simulink model "autocontroller_origin"  (R2024b)
settings: Solver=VariableStepAuto  StartTime=0.0  StopTime=10.0  RelTol=1e-3
undefined symbols (not defined in the file): control, controlParams, ControlSampleTime, Cruise_a, flightState, FWControlParams, FWTrimSpeed, uavParam, w_trim
libraries: slpidlib x21, simulink x8
(part 1 of 3)
settings Model: Creator=USER  LastModifiedBy=USER

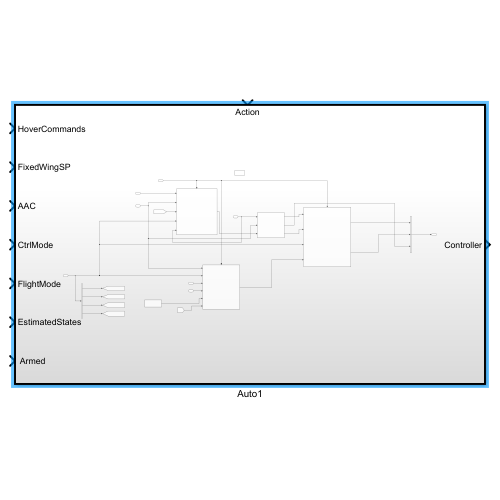
[thumbnail: Simulink's stored preview of the top-level diagram]
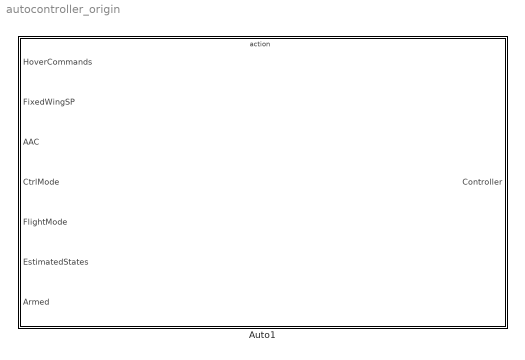
== system autocontroller_origin ==
  Auto1 : Subsystem  TreatAsAtomicUnit=on

== system autocontroller_origin/Auto1 ==
  HoverCommands : Inport  OutDataTypeStr=Bus: HoverSPBus
  FixedWingSP : Inport  Port=2
  AAC : Inport  Port=3
  CtrlMode : Inport  Port=4
  FlightMode : Inport  Port=5
  EstimatedStates : Inport  Port=6
  " Armed" : Inport  Port=7
  Action Port : ActionPort
  Blend Scheduler : Subsystem
  Bus Creator : BusCreator  Inputs=3  OutDataTypeStr=Bus: controller
  Bus Selector2 : BusSelector  OutputSignals=inTransition,TransitionCondition,BackTransitionCondition,TransitionStep
  Fixed Wing Controller : Subsystem  TreatAsAtomicUnit=on  VariantControl=Fixed Wing Controller
  Manual Control : Subsystem
  Multicopter Controller : Subsystem  TreatAsAtomicUnit=on
  Scheduler : Subsystem  SystemSampleTime=0.005
  Controller : Outport
  wires:
  Scheduler/1(MotorActuatorCommands) -> Bus Creator/1  "MotorActuatorCommands"
  Manual Control/1(AERT) -> Fixed Wing Controller/5(AERT)
  Scheduler/2(CtrlSurfaceCommands) -> Bus Creator/2  "CtrlSurfaceCommands"
  Fixed Wing Controller/1(Actuator) -> Scheduler/4(FixedWingActuators)
  Blend Scheduler/2(alpha) -> Bus Creator/3  "a"
  Multicopter Controller/1(MixerCommands) -> Blend Scheduler/3(MixerCommands)
  AAC/1 -> Fixed Wing Controller/3(AAC SP)
  FixedWingSP/1 -> Fixed Wing Controller/4(FixedWingSP)
  [InTransition] -> Multicopter Controller/3(InTransition)
  " Armed"/1 -> Fixed Wing Controller/Enable, Scheduler/Enable, Multicopter Controller/Enable
  HoverCommands/1 -> Multicopter Controller/1(Hover Commands)
  EstimatedStates/1 -> Fixed Wing Controller/1(States), Blend Scheduler/2(States), Multicopter Controller/2(States)
  FlightMode/1 -> Multicopter Controller/5(FlightMode), Blend Scheduler/1(FlightMode)
  Bus Selector2/2 -> [TransitionDone]  "<TransitionCondition>"
  CtrlMode/1 -> Bus Selector2/1, Scheduler/3(CtrlMode), Multicopter Controller/4(CtrlMode), Fixed Wing Controller/2(Control Mode)
  Bus Selector2/1 -> [InTransition]  "<inTransition>"
  Bus Selector2/3 -> [BackTransitionDone]  "<BackTransitionCondition>"
  Bus Creator/1 -> Controller/1
  Blend Scheduler/3(FlightState) -> Scheduler/2(FlightState)
  [InTransition] -> Fixed Wing Controller/6(In1)
  Bus Selector2/4 -> [TransitionStep]  "<TransitionStep>"
  Blend Scheduler/1(MotorCommands) -> Scheduler/1(MotorCommands)

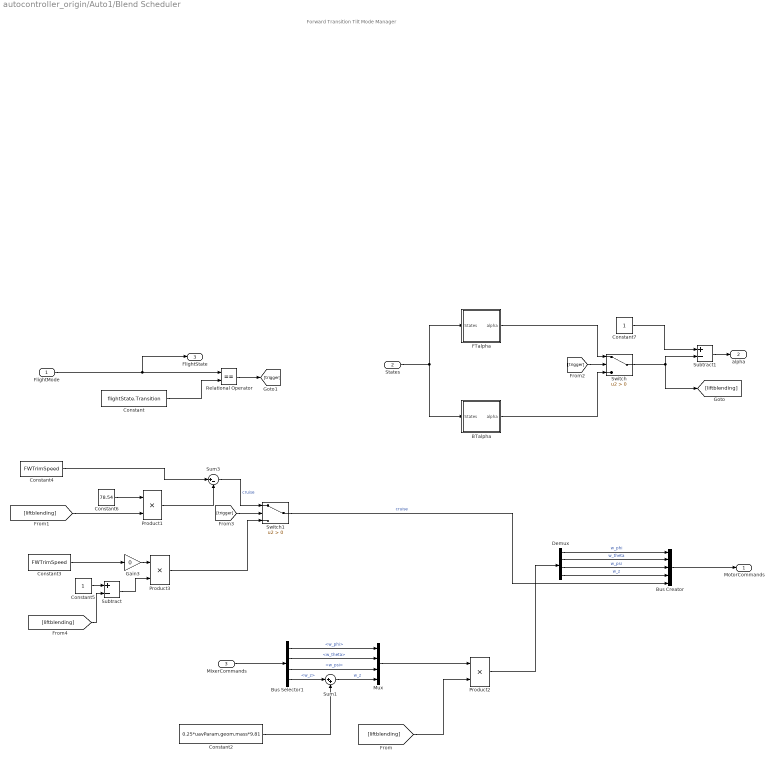
== system autocontroller_origin/Auto1/Blend Scheduler ==
  note: Forward Transition Tilt Mode Manager
  FlightMode : Inport
  States : Inport  Port=2
  MixerCommands : Inport  Port=3
  BTalpha : Subsystem  TreatAsAtomicUnit=on
  Bus Creator : BusCreator  Inputs=5
  Bus Selector1 : BusSelector  OutputSignals=w_phi,w_theta,w_psi,w_z
  Constant : Constant  Value=flightState.Transition
  Constant2 : Constant  Value=0.25*uavParam.geom.mass*9.81
  Constant3 : Constant  Value=FWTrimSpeed
  Constant4 : Constant  Value=FWTrimSpeed
  Constant5 : Constant
  Constant6 : Constant  Value=78.54
  Constant7 : Constant
  Demux : Demux
  FTalpha : Subsystem
  Gain3 : Gain  Gain=0
  Mux : Mux
  Product1 : Product
  Product2 : Product
  Product3 : Product
  Relational Operator : RelationalOperator  Operator===  OutDataTypeStr=boolean  RndMeth=Simplest  InputSameDT=off
  Subtract : Sum  Inputs=+-
  Subtract1 : Sum  Inputs=+-
  Sum1 : Sum  Inputs=|++
  Sum3 : Sum  Inputs=|+-
  Switch : Switch  Criteria=u2 > Threshold  SaturateOnIntegerOverflow=off  InputSameDT=off
  Switch1 : Switch  Criteria=u2 > Threshold  SaturateOnIntegerOverflow=off  InputSameDT=off
  MotorCommands : Outport
  alpha : Outport  Port=2
  FlightState : Outport  Port=3
  wires:
  FlightMode/1 -> Relational Operator/1, FlightState/1
  Relational Operator/1 -> [trigger]
  Bus Selector1/4 -> Sum1/1  "<w_z>"
  Constant2/1 -> Sum1/2
  [liftblending] -> Product2/2
  Mux/1 -> Product2/1
  MixerCommands/1 -> Bus Selector1/1
  Bus Selector1/1 -> Mux/1  "<w_phi>"
  Bus Selector1/2 -> Mux/2  "<w_theta>"
  Bus Selector1/3 -> Mux/3  "<w_psi>"
  Sum1/1 -> Mux/4  "w_z"
  Product2/1 -> Demux/1
  Demux/1 -> Bus Creator/1  "w_phi"
  Demux/2 -> Bus Creator/2  "w_theta"
  Demux/3 -> Bus Creator/3  "w_psi"
  Demux/4 -> Bus Creator/4  "w_z"
  Bus Creator/1 -> MotorCommands/1
  Constant6/1 -> Product1/1
  States/1 -> FTalpha/1(States), BTalpha/1(States)
  Switch/1 -> [liftblending], Subtract1/2
  FTalpha/1(alpha) -> Switch/1
  BTalpha/1(alpha) -> Switch/3
  [trigger] -> Switch/2
  Product1/1 -> Sum3/2
  Sum3/1 -> Switch1/1  "cruise"
  [trigger] -> Switch1/2
  Switch1/1 -> Bus Creator/5  "cruise"
  Constant3/1 -> Gain3/1
  Gain3/1 -> Product3/1
  Constant5/1 -> Subtract/1
  [liftblending] -> Subtract/2
  Subtract/1 -> Product3/2
  Product3/1 -> Switch1/3
  Constant7/1 -> Subtract1/1
  Subtract1/1 -> alpha/1
  Constant/1 -> Relational Operator/2
  [liftblending] -> Product1/2
  Constant4/1 -> Sum3/1

== system autocontroller_origin/Auto1/Fixed Wing Controller ==
  States : Inport
  Control Mode : Inport  Port=2
  AAC SP : Inport  Port=3  OutDataTypeStr=Bus: AAC
  FixedWingSP : Inport  Port=4  OutDataTypeStr=Bus: FixedWingCommandBus
  AERT : Inport  Port=5
  In1 : Inport  Port=6
  Actuator Armed : EnablePort
  Subsystem : Subsystem
  Actuator : Outport
  wires:
  States/1 -> Subsystem/1(States)
  Control Mode/1 -> Subsystem/2(Control Mode)
  AAC SP/1 -> Subsystem/3(AAC SP)
  Subsystem/1(Actuator) -> Actuator/1
  AERT/1 -> Subsystem/5(AERT)
  FixedWingSP/1 -> Subsystem/4(FixedWingSP)
  In1/1 -> Subsystem/6(Intransition)

== system autocontroller_origin/Auto1/Manual Control ==
  Bus Creator : BusCreator  Inputs=4
  Constant{,1..3} (4 alike) : Constant  Value=0  SampleTime=-1
  AERT : Outport
  wires:
  Constant/1 -> Bus Creator/1  "aileron"
  Constant1/1 -> Bus Creator/2  "throttle"
  Constant2/1 -> Bus Creator/3  "elevator"
  Constant3/1 -> Bus Creator/4  "rudder"
  Bus Creator/1 -> AERT/1

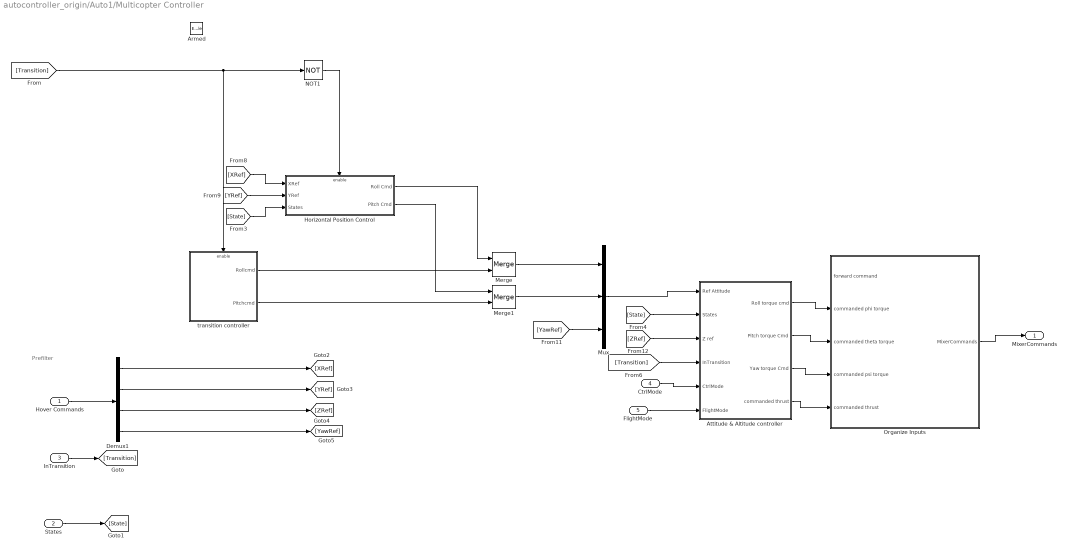
== system autocontroller_origin/Auto1/Multicopter Controller ==
  note: Prefilter
  Hover Commands : Inport  OutDataTypeStr=Bus: HoverSPBus
  States : Inport  Port=2
  InTransition : Inport  Port=3
  CtrlMode : Inport  Port=4
  FlightMode : Inport  Port=5
  " Armed" : EnablePort
  Attitude & Altitude controller : Subsystem
  Demux1 : Demux
  Horizontal Position Control : Subsystem  TreatAsAtomicUnit=on
  Merge : Merge
  Merge1 : Merge
  Mux : Mux  Inputs=3
  NOT1 : Logic  Operator=NOT  IconShape=distinctive  AllPortsSameDT=off  OutDataTypeStr=boolean
  Organize Inputs : Subsystem
  transition controller : Subsystem
  MixerCommands : Outport
  wires:
  Organize Inputs/1(MixerCommands) -> MixerCommands/1
  Demux1/1 -> [XRef]
  [State] -> Horizontal Position Control/3(States)
  Demux1/3 -> [ZRef]
  NOT1/1 -> Horizontal Position Control/Enable
  [XRef] -> Horizontal Position Control/1(XRef)
  [YRef] -> Horizontal Position Control/2(YRef)
  InTransition/1 -> [Transition]
  States/1 -> [State]
  Hover Commands/1 -> Demux1/1
  Demux1/4 -> [YawRef]
  Mux/1 -> Attitude & Altitude controller/1(Ref Attitude)
  [State] -> Attitude & Altitude controller/2(States)
  [ZRef] -> Attitude & Altitude controller/3(Z ref)
  [Transition] -> Attitude & Altitude controller/4(InTransition)
  Attitude & Altitude controller/1(Roll torque cmd) -> Organize Inputs/2(commanded phi torque)
  Attitude & Altitude controller/2(Pitch torque Cmd) -> Organize Inputs/3(commanded theta torque)
  Attitude & Altitude controller/4(commanded thrust) -> Organize Inputs/5(commanded thrust)
  FlightMode/1 -> Attitude & Altitude controller/6(FlightMode)
  Attitude & Altitude controller/3(Yaw torque Cmd) -> Organize Inputs/4(commanded psi torque)
  [Transition] -> NOT1/1, transition controller/Enable
  [YawRef] -> Mux/3
  Demux1/2 -> [YRef]
  Merge/1 -> Mux/1
  Merge1/1 -> Mux/2
  transition controller/1(Rollcmd) -> Merge/2
  transition controller/2(Pitchcmd) -> Merge1/2
  Horizontal Position Control/1(Roll Cmd) -> Merge/1
  Horizontal Position Control/2(Pitch Cmd) -> Merge1/1
  CtrlMode/1 -> Attitude & Altitude controller/5(CtrlMode)

== system autocontroller_origin/Auto1/Scheduler ==
  MotorCommands : Inport
  FlightState : Inport  Port=2  OutDataTypeStr=Enum: flightState
  CtrlMode : Inport  Port=3
  FixedWingActuators : Inport  Port=4
  " Armed" : EnablePort
  FixedWingScheduler : Subsystem
  Subsystem : Subsystem
  MotorActuatorCommands : Outport  OutputWhenDisabled=reset  InitialOutput=0
  CtrlSurfaceCommands : Outport  Port=2  OutDataTypeStr=Bus: FixedWingCtrlBus  OutputWhenDisabled=reset  InitialOutput=0  VectorParamsAs1DForOutWhenUnconnected=off
  wires:
  FixedWingScheduler/1(ActuatorControls) -> CtrlSurfaceCommands/1, Subsystem/2(FixedWingActuators)
  FlightState/1 -> Subsystem/1(FlightState), FixedWingScheduler/1(FlightState)
  Subsystem/1(ActuatorControls) -> MotorActuatorCommands/1
  MotorCommands/1 -> Subsystem/4(MotorCommands)
  FixedWingActuators/1 -> FixedWingScheduler/2(FixedWingActuators)
  CtrlMode/1 -> Subsystem/3(CtrlMode)

== system autocontroller_origin/Auto1/Blend Scheduler/BTalpha ==
  States : Inport
  Bus Selector : BusSelector  OutputSignals=airspeed
  Constant : Constant  Value=65
  Gain : Gain  Gain=1/20
  Saturation : Saturate  UpperLimit=1  LowerLimit=0
  Subtract : Sum  Inputs=+-
  alpha : Outport
  wires:
  Constant/1 -> Subtract/1
  Subtract/1 -> Gain/1
  Gain/1 -> Saturation/1
  Saturation/1 -> alpha/1
  States/1 -> Bus Selector/1
  Bus Selector/1 -> Subtract/2  "<airspeed>"

== system autocontroller_origin/Auto1/Blend Scheduler/FTalpha ==
  States : Inport
  1-a : Sum  Inputs=+-
  Bus Selector : BusSelector  OutputSignals=airspeed
  Constant3 : Constant  Value=35
  Constant5 : Constant  Value=Cruise_a
  Gain3 : Gain  Gain=1/10
  Saturation1 : Saturate  UpperLimit=10  LowerLimit=0
  Sum2 : Sum  Inputs=|+-
  alpha : Outport
  wires:
  1-a/1 -> alpha/1
  Bus Selector/1 -> Sum2/1  "<airspeed>"
  Gain3/1 -> 1-a/2
  Sum2/1 -> Saturation1/1
  Saturation1/1 -> Gain3/1
  Constant3/1 -> Sum2/2
  States/1 -> Bus Selector/1
  Constant5/1 -> 1-a/1

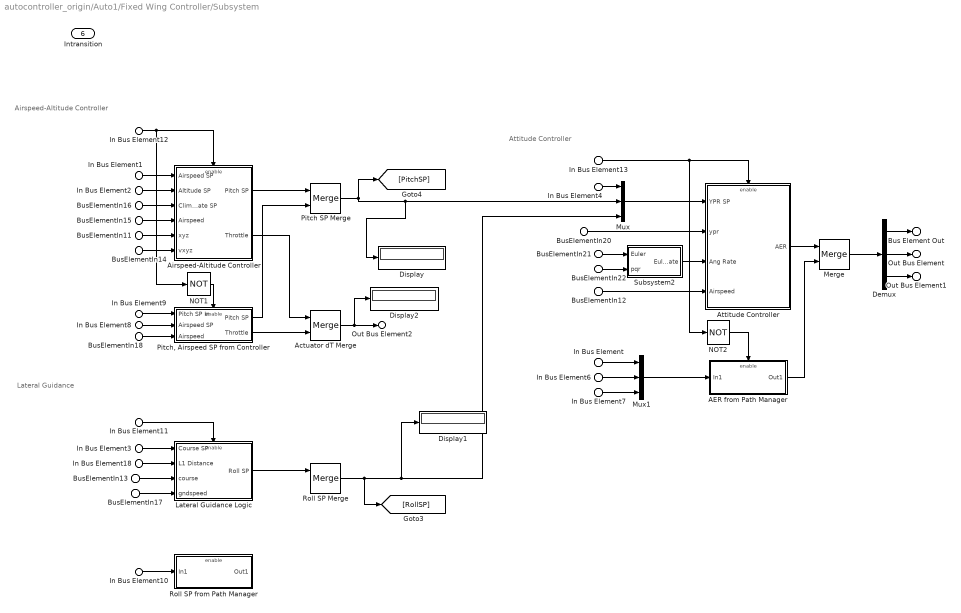
== system autocontroller_origin/Auto1/Fixed Wing Controller/Subsystem ==
  note: Airspeed-Altitude Controller
  note: Lateral Guidance
  note: Attitude Controller
  BusElementIn11 : Inport  PortName=States  Element=Xe
  BusElementIn12 : Inport  PortName=States  Element=airspeed
  BusElementIn15 : Inport  PortName=States  Element=airspeed
  BusElementIn18 : Inport  PortName=States  Element=airspeed
  BusElementIn13 : Inport  PortName=States  Element=course
  BusElementIn16 : Inport  PortName=States  Element=course
  BusElementIn14 : Inport  PortName=States  Element=Ve_ground
  BusElementIn17 : Inport  PortName=States  Element=gndspeed
  BusElementIn20 : Inport  PortName=States  Element=YPR
  BusElementIn21 : Inport  PortName=States  Element=Euler
  BusElementIn22 : Inport  PortName=States  Element=pqr
  In Bus Element11 : Inport  Port=2  PortName=Control Mode  Element=lateralGuidance
  In Bus Element12 : Inport  Port=2  PortName=Control Mode  Element=airspeedAltitude
  In Bus Element13 : Inport  Port=2  PortName=Control Mode  Element=attitude
  In Bus Element1 : Inport  Port=3  PortName=AAC SP  Element=airspeed
  In Bus Element2 : Inport  Port=3  PortName=AAC SP  Element=altitude
  In Bus Element18 : Inport  Port=3  PortName=AAC SP  Element=L1
  In Bus Element3 : Inport  Port=3  PortName=AAC SP  Element=course
  In Bus Element4 : Inport  Port=4  PortName=FixedWingSP  Element=yaw
  In Bus Element9 : Inport  Port=4  PortName=FixedWingSP  Element=pitch
  In Bus Element10 : Inport  Port=4  PortName=FixedWingSP  Element=roll
  In Bus Element8 : Inport  Port=4  PortName=FixedWingSP  Element=airspeed
  In Bus Element : Inport  Port=5  PortName=AERT  Element=aileron
  In Bus Element6 : Inport  Port=5  PortName=AERT  Element=elevator
  In Bus Element7 : Inport  Port=5  PortName=AERT  Element=rudder
  Intransition : Inport  Port=6
  AER from Path Manager : Subsystem  TreatAsAtomicUnit=on
  Actuator dT Merge : Merge
  Airspeed-Altitude Controller : Subsystem
  Attitude Controller : Subsystem
  Demux : Demux  Outputs=3
  Display : Display
  Display1 : Display
  Display2 : Display
  Lateral Guidance Logic : Subsystem
  Merge : Merge
  Mux : Mux  Inputs=3
  Mux1 : Mux  Inputs=3
  NOT1 : Logic  Operator=NOT  IconShape=distinctive  AllPortsSameDT=off  OutDataTypeStr=boolean
  NOT2 : Logic  Operator=NOT  IconShape=distinctive  AllPortsSameDT=off  OutDataTypeStr=boolean
  Pitch SP Merge : Merge
  "Pitch, Airspeed SP from Controller" : Subsystem  TreatAsAtomicUnit=on
  Roll SP Merge : Merge
  Roll SP from Path Manager : Subsystem  TreatAsAtomicUnit=on
  Subsystem2 : Subsystem
  Bus Element Out : Outport  PortName=Actuator  Element=dA
  Out Bus Element : Outport  PortName=Actuator  Element=dE
  Out Bus Element1 : Outport  PortName=Actuator  Element=dR
  Out Bus Element2 : Outport  PortName=Actuator  Element=dT
  wires:
  In Bus Element4/1 -> Mux/1
  Roll SP Merge/1 -> [RollSP], Display1/1, Mux/3
  BusElementIn18/1 -> "Pitch, Airspeed SP from Controller"/3(Airspeed)
  In Bus Element12/1 -> Airspeed-Altitude Controller/Enable, NOT1/1
  In Bus Element3/1 -> Lateral Guidance Logic/1(Course SP)
  Mux1/1 -> AER from Path Manager/1(In1)
  In Bus Element11/1 -> Lateral Guidance Logic/Enable
  Lateral Guidance Logic/1(Roll SP) -> Roll SP Merge/1
  In Bus Element7/1 -> Mux1/3
  Demux/2 -> Out Bus Element/1
  Demux/1 -> Bus Element Out/1
  In Bus Element9/1 -> "Pitch, Airspeed SP from Controller"/1(Pitch SP In)
  Merge/1 -> Demux/1
  In Bus Element18/1 -> Lateral Guidance Logic/2(L1 Distance)
  In Bus Element13/1 -> NOT2/1, Attitude Controller/Enable
  "Pitch, Airspeed SP from Controller"/1(Pitch SP) -> Pitch SP Merge/2
  BusElementIn14/1 -> Airspeed-Altitude Controller/6(vxyz)
  Pitch SP Merge/1 -> Display/1, Mux/2, [PitchSP]
  BusElementIn15/1 -> Airspeed-Altitude Controller/4(Airspeed)
  In Bus Element8/1 -> "Pitch, Airspeed SP from Controller"/2(Airspeed SP)
  BusElementIn13/1 -> Lateral Guidance Logic/3(course)
  Airspeed-Altitude Controller/2(Throttle) -> Actuator dT Merge/1
  BusElementIn16/1 -> Airspeed-Altitude Controller/3(Climb Rate SP)
  In Bus Element1/1 -> Airspeed-Altitude Controller/1(Airspeed SP)
  BusElementIn11/1 -> Airspeed-Altitude Controller/5(xyz)
  BusElementIn12/1 -> Attitude Controller/4(Airspeed)
  In Bus Element2/1 -> Airspeed-Altitude Controller/2(Altitude SP)
  BusElementIn20/1 -> Attitude Controller/2(ypr)
  Mux/1 -> Attitude Controller/1(YPR SP)
  Demux/3 -> Out Bus Element1/1
  BusElementIn21/1 -> Subsystem2/1(Euler)
  Subsystem2/1(Euler Rate) -> Attitude Controller/3(Ang Rate)
  "Pitch, Airspeed SP from Controller"/2(Throttle) -> Actuator dT Merge/2
  Airspeed-Altitude Controller/1(Pitch SP) -> Pitch SP Merge/1
  Attitude Controller/1(AER) -> Merge/1
  AER from Path Manager/1(Out1) -> Merge/2
  In Bus Element/1 -> Mux1/1
  In Bus Element10/1 -> Roll SP from Path Manager/1(In1)
  In Bus Element6/1 -> Mux1/2
  NOT2/1 -> AER from Path Manager/Enable
  BusElementIn22/1 -> Subsystem2/2(pqr)
  Actuator dT Merge/1 -> Display2/1, Out Bus Element2/1
  BusElementIn17/1 -> Lateral Guidance Logic/4(gndspeed)
  NOT1/1 -> "Pitch, Airspeed SP from Controller"/Enable

== system autocontroller_origin/Auto1/Multicopter Controller/Attitude & Altitude controller ==
  Ref Attitude : Inport
  States : Inport  Port=2
  Z ref : Inport  Port=3
  InTransition : Inport  Port=4
  CtrlMode : Inport  Port=5
  FlightMode : Inport  Port=6
  Altitude Control : Subsystem
  Bus Selector : BusSelector  OutputSignals=RC
  Compare To Constant : simulink/Logic and Bit Operations/Compare To Constant  relop=>  const=1700  OutDataTypeStr=boolean
  Derivative Gain : Subsystem  VariantControl=AttitudeControl==1
  Selector : Selector  InputPortWidth=10  IndexOptions=Index vector (dialog)  Indices=7  OutputSizes=1
  Roll torque cmd : Outport
  Pitch torque Cmd : Outport  Port=2
  Yaw torque Cmd : Outport  Port=3
  commanded thrust : Outport  Port=4
  wires:
  Altitude Control/1(commanded thrust) -> commanded thrust/1
  Derivative Gain/1(Roll torque cmd) -> Roll torque cmd/1
  InTransition/1 -> Altitude Control/3(InTransition)
  Derivative Gain/2(Pitch torque Cmd) -> Pitch torque Cmd/1
  States/1 -> Derivative Gain/2(States), Bus Selector/1, Altitude Control/1(States)
  Derivative Gain/3(Yaw torque Cmd) -> Yaw torque Cmd/1
  Z ref/1 -> Altitude Control/2(Z ref)
  FlightMode/1 -> Altitude Control/4(FlightMode)
  Ref Attitude/1 -> Derivative Gain/1(Ref Attitude)
  Selector/1 -> Compare To Constant/1
  Bus Selector/1 -> Selector/1  "<RC>"
  Compare To Constant/1 -> Altitude Control/Enable
  CtrlMode/1 -> Derivative Gain/3(CtrlMode), Altitude Control/5(CtrlMode)

== system autocontroller_origin/Auto1/Multicopter Controller/Horizontal Position Control ==
  note: Forward Motion is controlled using Tilt.
      | Lateral Motion occurs using roll.
  XRef : Inport
  YRef : Inport  Port=2
  States : Inport  Port=3
  Enable : EnablePort  ShowOutputPort=on
  Saturation : Saturate  UpperLimit=0.75  LowerLimit=-0.75
  Saturation1 : Saturate  UpperLimit=1  LowerLimit=-0.75
  Signal Conversion : SignalConversion  OverrideOpt=off
  Signal Conversion1 : SignalConversion  OverrideOpt=off
  XY Controller : Subsystem
  Roll Cmd : Outport
  Pitch Cmd : Outport  Port=2
  wires:
  XRef/1 -> XY Controller/1(X_ref)
  YRef/1 -> XY Controller/2(Y_ref)
  States/1 -> XY Controller/3(States)
  XY Controller/1(Forward cmd) -> Saturation1/1
  XY Controller/2(Sideward Cmd) -> Saturation/1
  Saturation1/1 -> Signal Conversion/1
  Saturation/1 -> Signal Conversion1/1
  Signal Conversion/1 -> Pitch Cmd/1
  Signal Conversion1/1 -> Roll Cmd/1
  Enable/1 -> XY Controller/Enable

== system autocontroller_origin/Auto1/Multicopter Controller/Organize Inputs ==
  forward command : Inport
  commanded phi torque : Inport  Port=2
  commanded theta torque : Inport  Port=3
  commanded psi torque : Inport  Port=4
  commanded thrust : Inport  Port=5
  Out Bus Element : Outport  PortName=MixerCommands  Element=w_phi
  Out Bus Element1 : Outport  PortName=MixerCommands  Element=w_theta
  Out Bus Element2 : Outport  PortName=MixerCommands  Element=w_psi
  Out Bus Element3 : Outport  PortName=MixerCommands  Element=w_z
  Out Bus Element4 : Outport  PortName=MixerCommands  Element=l_x
  wires:
  forward command/1 -> Out Bus Element4/1
  commanded phi torque/1 -> Out Bus Element/1  "phi"
  commanded theta torque/1 -> Out Bus Element1/1
  commanded psi torque/1 -> Out Bus Element2/1
  commanded thrust/1 -> Out Bus Element3/1

== system autocontroller_origin/Auto1/Multicopter Controller/transition controller ==
  Enable : EnablePort
  Constant : Constant  Value=0
  Constant1 : Constant  Value=0
  Rollcmd : Outport
  Pitchcmd : Outport  Port=2
  wires:
  Constant/1 -> Rollcmd/1
  Constant1/1 -> Pitchcmd/1

== system autocontroller_origin/Auto1/Scheduler/FixedWingScheduler ==
  note: C opyright 2024 The MathWorks, Inc.
  note: Fixed Wing Control Mixer
  FlightState : Inport
  FixedWingActuators : Inport  Port=2  OutDataTypeStr=Bus: FixedWingCtrlBus
  Merge : Merge  Inputs=4
  Switch Case : SwitchCase  CaseConditions={flightState.Hover, flightState.Transition, flightState.FixedWing,flightState.BackTransition}  ShowDefaultCase=off
  Switch Case Action Subsystem : Subsystem  TreatAsAtomicUnit=on
  Switch Case Action Subsystem1 : Subsystem  TreatAsAtomicUnit=on
  Switch Case Action Subsystem2 : Subsystem  TreatAsAtomicUnit=on
  Switch Case Action Subsystem3 : Subsystem  TreatAsAtomicUnit=on
  ActuatorControls : Outport
  wires:
  FlightState/1 -> Switch Case/1
  FixedWingActuators/1 -> Switch Case Action Subsystem2/1(FixedWingActuators), Switch Case Action Subsystem1/1(FixedWingActuators)
  Switch Case/3 -> Switch Case Action Subsystem2/Action
  Switch Case/2 -> Switch Case Action Subsystem1/Action
  Switch Case Action Subsystem3/1(FixedWingControls) -> Merge/4
  Merge/1 -> ActuatorControls/1
  Switch Case Action Subsystem1/1(FixedWingControls) -> Merge/2
  Switch Case/4 -> Switch Case Action Subsystem3/Action
  Switch Case Action Subsystem/1(FixedWingControls) -> Merge/1
  Switch Case/1 -> Switch Case Action Subsystem/Action
  Switch Case Action Subsystem2/1(FixedWingControls) -> Merge/3

== system autocontroller_origin/Auto1/Scheduler/Subsystem ==
  note: C opyright 2024 The MathWorks, Inc.
  note: Multicopter Control Mixer
  FlightState : Inport
  FixedWingActuators : Inport  Port=2
  CtrlMode : Inport  Port=3
  MotorCommands : Inport  Port=4
  Actuator To Voltage : Subsystem
  Merge : Merge  Inputs=4
  Switch Case : SwitchCase  CaseConditions={flightState.Hover, flightState.Transition, flightState.FixedWing,flightState.BackTransition}  ShowDefaultCase=off
  Switch Case Action Subsystem : Subsystem  TreatAsAtomicUnit=on
  Switch Case Action Subsystem1 : Subsystem  TreatAsAtomicUnit=on
  Switch Case Action Subsystem2 : Subsystem  TreatAsAtomicUnit=on
  Switch Case Action Subsystem3 : Subsystem  TreatAsAtomicUnit=on
  ActuatorControls : Outport  OutDataTypeStr=Bus: FCCData
  wires:
  Switch Case/4 -> Switch Case Action Subsystem3/Action
  MotorCommands/1 -> Switch Case Action Subsystem3/1(MixerCommands), Switch Case Action Subsystem/1(MixerCommands), Switch Case Action Subsystem1/1(MixerCommands)
  FlightState/1 -> Switch Case/1
  Switch Case Action Subsystem3/1(Actuator) -> Merge/4
  FixedWingActuators/1 -> Switch Case Action Subsystem2/1(FixedWingCtrlBus)
  Switch Case/3 -> Switch Case Action Subsystem2/Action
  Switch Case/2 -> Switch Case Action Subsystem1/Action
  Switch Case Action Subsystem1/1(Actuator) -> Merge/2
  Switch Case/1 -> Switch Case Action Subsystem/Action
  Switch Case Action Subsystem2/1(Actuator) -> Merge/3
  Switch Case Action Subsystem/1(Actuator) -> Merge/1
  Merge/1 -> Actuator To Voltage/2(Motor Commands)
  Actuator To Voltage/1(Actuator) -> ActuatorControls/1
  CtrlMode/1 -> Actuator To Voltage/1(CtrlMode)

== system autocontroller_origin/Auto1/Fixed Wing Controller/Subsystem/AER from Path Manager ==
  In1 : Inport
  Enable : EnablePort
  Out1 : Outport
  wires:
  In1/1 -> Out1/1

== system autocontroller_origin/Auto1/Fixed Wing Controller/Subsystem/Airspeed-Altitude Controller ==
  note: Airspeed and altitude are controlled independently
      | by ignoring their coupled dynamics.
  Airspeed SP : Inport
  Altitude SP : Inport  Port=2
  Climb Rate SP : Inport  Port=3
  Airspeed : Inport  Port=4
  xyz : Inport  Port=5
  vxyz : Inport  Port=6
  Control Mode : EnablePort  ShowOutputPort=on
  Airspeed Controller : slpidlib/PID Controller  Controller=PID  Form=Parallel  TimeDomain=Discrete-time  UseExternalTs=off  SampleTime=ControlSampleTime  IntegratorMethod=Trapezoidal  FilterMethod=Forward Euler  ControllerParametersSource=internal  P=FWControlParams.P_AIRSPD  I=FWControlParams.I_AIRSPD  UseKiTs=off  D=FWControlParams.D_AIRSPD  UseExternalDerivativeSource=off  N=FWControlParams.N_AIRSPD  UseFilter=on  TunerSelectOption=Transfer Function Based (PID Tuner App)  InitialConditionSource=internal  InitialConditionForIntegrator=0  InitialConditionForFilter=0  DifferentiatorICPrevScaledInput=0  ExternalReset=none  TrackingMode=off  Kt=1  LimitOutput=off  SatLimitsSource=internal  UpperSaturationLimit=Inf  LowerSaturationLimit=0  LinearizeAsGain=on  AntiWindupMode=clamping  Kb=1  LimitIntegrator=off  UpperIntegratorSaturationLimit=inf  LowerIntegratorSaturationLimit=-inf  POutMin=[]  POutMax=[]  IOutMin=[]  IOutMax=[]  DOutMin=[]  DOutMax=[]  NOutMin=[]  NOutMax=[]  SumOutMin=[]  SumOutMax=[]  SaturationOutMin=[]  SaturationOutMax=[]  PParamMin=[]  PParamMax=[]  IParamMin=[]  IParamMax=[]  DParamMin=[]  DParamMax=[]  NParamMin=[]  NParamMax=[]  KbParamMin=[]  KbParamMax=[]  KtParamMin=[]  KtParamMax=[]  KbOutMin=[]  KbOutMax=[]  KtOutMin=[]  KtOutMax=[]  IntegratorOutMin=[]  IntegratorOutMax=[]  FilterOutMin=[]  FilterOutMax=[]  SumI1OutMin=[]  SumI1OutMax=[]  SumI2OutMin=[]  SumI2OutMax=[]  SumI3OutMin=[]  SumI3OutMax=[]  SumI4OutMin=[]  SumI4OutMax=[]  SumDOutMin=[]  SumDOutMax=[]  DifferentiatorOutMin=[]  DifferentiatorOutMax=[]  FilterDiffOutCoefMin=[]  FilterDiffOutCoefMax=[]  ReciprocalOutMin=[]  ReciprocalOutMax=[]  SumDenOutMin=[]  SumDenOutMax=[]  SumNumOutMin=[]  SumNumOutMax=[]  DivideOutMin=[]  DivideOutMax=[]  UdiffTsProdOutMin=[]  UdiffTsProdOutMax=[]  NTsProdOutMin=[]  NTsProdOutMax=[]  UintegralTsProdOutMin=[]  UintegralTsProdOutMax=[]  UngainTsProdOutMin=[]  UngainTsProdOutMax=[]  ClampingZeroOutDataTypeStr=Inherit: Inherit via back propagation  ClampingZeroOutMin=[]  ClampingZeroOutMax=[]  FilterDenConstantOutDataTypeStr=Inherit: Inherit via back propagation  FilterDenConstantOutMin=[]  FilterDenConstantOutMax=[]  PCopyOutDataTypeStr=Inherit: Inherit via back propagation  PCopyOutMin=[]  PCopyOutMax=[]  NCopyOutDataTypeStr=Inherit: Inherit via back propagation  NCopyOutMin=[]  NCopyOutMax=[]  IntegratorContinuousStateAttributes=''  IntegratorStateMustResolveToSignalObject=off  IntegratorRTWStateStorageClass=Auto  FilterContinuousStateAttributes=''  FilterStateMustResolveToSignalObject=off  FilterRTWStateStorageClass=Auto  ParallelPVariant=InternalParameters  IdealPVariant=Disabled  IVariant=InternalParameters  DVariant=InternalParameters  IntegratorVariant=Discrete  SatVariant=Disabled  AWVariant=Passthrough  PCopyVariant=Disabled  TRVariant=Disabled  FdbkBlocksVariant=Forward  IdealPFdbkVariant=Disabled  SatFdbkVariant=Disabled  DerivativeFilterVariant=ForwardEulerFilter  NVariant=InternalParameters  NCopyVariant=Disabled  FilterICVariant=InternalICsFilter  IntegratorICVariant=InternalICs  ExternalResetVariant=Disabled  TRSumVariant=Passthrough  SumFdbkVariant=Disabled  SumVariant=Sum_PID  TsampFilterVariant=InternalTs  TsampNgainVariant=Passthrough  TsampIntegralVariant=Disabled_SignalSpec  ExternalSaturationOutDataTypeStr=Inherit: Same as second input  DerivativeSourceVariant=ErrorSignal  PreIntVariant=InternalPreInt
  Altitude controller : Subsystem
  Climb Rate SP Merge : Merge
  Climb Rate SP from Guidance : Subsystem  TreatAsAtomicUnit=on
  Compare To Constant : simulink/Logic and Bit Operations/Compare To Constant  relop===  const=uint8(1)  OutDataTypeStr=boolean
  Compare To Constant1 : simulink/Logic and Bit Operations/Compare To Constant  relop===  const=uint8(2)  OutDataTypeStr=boolean
  Pitch SP Controller : Subsystem
  Sum1 : Sum  Inputs=|+-
  Pitch SP : Outport
  Throttle : Outport  Port=2
  wires:
  Airspeed SP/1 -> Sum1/1
  Sum1/1 -> Airspeed Controller/1
  Airspeed/1 -> Sum1/2
  Airspeed Controller/1 -> Throttle/1
  Altitude SP/1 -> Altitude controller/1(Alt SP)
  xyz/1 -> Altitude controller/2(xyz)
  vxyz/1 -> Pitch SP Controller/2(vxyz)
  Pitch SP Controller/1(Pitch SP) -> Pitch SP/1
  Control Mode/1 -> Compare To Constant1/1, Compare To Constant/1
  Compare To Constant/1 -> Altitude controller/Enable
  Compare To Constant1/1 -> Climb Rate SP from Guidance/Enable
  Altitude controller/1(Climb Rate SP) -> Climb Rate SP Merge/1
  Climb Rate SP from Guidance/1(Out1) -> Climb Rate SP Merge/2
  Climb Rate SP Merge/1 -> Pitch SP Controller/1(Climb Rate SP)
  Climb Rate SP/1 -> Climb Rate SP from Guidance/1(Climb Rate SP)

== system autocontroller_origin/Auto1/Fixed Wing Controller/Subsystem/Attitude Controller ==
  YPR SP : Inport
  ypr : Inport  Port=2
  Ang Rate : Inport  Port=3
  Airspeed : Inport  Port=4
  Enable : EnablePort  ShowOutputPort=on
  AER Merge : Merge
  Compare To Constant : simulink/Logic and Bit Operations/Compare To Constant  relop===  const=uint8(1)  OutDataTypeStr=boolean
  Compare To Constant1 : simulink/Logic and Bit Operations/Compare To Constant  relop===  const=uint8(2)  OutDataTypeStr=boolean
  Demux1 : Demux  Outputs=3
  Pitch Roll Controller : Subsystem
  Rudder Heading Controller : Subsystem
  AER : Outport
  wires:
  ypr/1 -> Rudder Heading Controller/2(YPR), Pitch Roll Controller/3(YPR)
  YPR SP/1 -> Demux1/1
  Enable/1 -> Compare To Constant1/1, Compare To Constant/1
  AER Merge/1 -> AER/1
  Compare To Constant/1 -> Pitch Roll Controller/Enable
  Pitch Roll Controller/1(AER) -> AER Merge/1
  Rudder Heading Controller/1(AER) -> AER Merge/2
  Demux1/1 -> Rudder Heading Controller/1(Yaw SP)
  Demux1/2 -> Pitch Roll Controller/1(Pitch SP)
  Demux1/3 -> Pitch Roll Controller/2(Roll SP)
  Ang Rate/1 -> Rudder Heading Controller/3(Ang Rate), Pitch Roll Controller/4(Ang Rate)
  Compare To Constant1/1 -> Rudder Heading Controller/Enable
  Airspeed/1 -> Pitch Roll Controller/5(Airspeed)

== system autocontroller_origin/Auto1/Fixed Wing Controller/Subsystem/Lateral Guidance Logic ==
  note: S. Park, J. Deyst, and J. P. How, "A New Nonlinear Guidance Logic for Trajectory Tracking," Proceedings of the AIAA Guidance, Navigation and Control Conference, Aug 2004. AIAA-2004-4900.
  Course SP : Inport
  L1 Distance : Inport  Port=2
  course : Inport  Port=3
  gndspeed : Inport  Port=4
  Enable : EnablePort
  Display{,1..3} (4 alike) : Display
  MATLAB Function : MATLAB Function  TreatAsAtomicUnit=on  SystemSampleTime=ControlSampleTime
  Terminator : Terminator
  Roll SP : Outport
  wires:
  course/1 -> Display1/1, MATLAB Function/2(course)
  MATLAB Function/2(rollSP) -> Roll SP/1
  MATLAB Function/1(lacc) -> Terminator/1
  gndspeed/1 -> Display2/1, MATLAB Function/3(groundSpeed)
  L1 Distance/1 -> Display3/1, MATLAB Function/4(L1)
  Course SP/1 -> Display/1, MATLAB Function/1(courseSP)

== system autocontroller_origin/Auto1/Fixed Wing Controller/Subsystem/Pitch, Airspeed SP from Controller ==
  Pitch SP In : Inport
  Airspeed SP : Inport  Port=2
  Airspeed : Inport  Port=3
  Enable : EnablePort
  Airspeed Controller : slpidlib/PID Controller  Controller=PID  Form=Parallel  TimeDomain=Discrete-time  UseExternalTs=off  SampleTime=ControlSampleTime  IntegratorMethod=Trapezoidal  FilterMethod=Forward Euler  ControllerParametersSource=internal  P=FWControlParams.P_AIRSPD  I=FWControlParams.I_AIRSPD*0  UseKiTs=off  D=FWControlParams.D_AIRSPD*0  UseExternalDerivativeSource=off  N=FWControlParams.N_AIRSPD  UseFilter=on  TunerSelectOption=Transfer Function Based (PID Tuner App)  InitialConditionSource=internal  InitialConditionForIntegrator=0  InitialConditionForFilter=0  DifferentiatorICPrevScaledInput=0  ExternalReset=none  TrackingMode=off  Kt=1  LimitOutput=off  SatLimitsSource=internal  UpperSaturationLimit=Inf  LowerSaturationLimit=0  LinearizeAsGain=on  AntiWindupMode=clamping  Kb=1  LimitIntegrator=off  UpperIntegratorSaturationLimit=inf  LowerIntegratorSaturationLimit=-inf  POutMin=[]  POutMax=[]  IOutMin=[]  IOutMax=[]  DOutMin=[]  DOutMax=[]  NOutMin=[]  NOutMax=[]  SumOutMin=[]  SumOutMax=[]  SaturationOutMin=[]  SaturationOutMax=[]  PParamMin=[]  PParamMax=[]  IParamMin=[]  IParamMax=[]  DParamMin=[]  DParamMax=[]  NParamMin=[]  NParamMax=[]  KbParamMin=[]  KbParamMax=[]  KtParamMin=[]  KtParamMax=[]  KbOutMin=[]  KbOutMax=[]  KtOutMin=[]  KtOutMax=[]  IntegratorOutMin=[]  IntegratorOutMax=[]  FilterOutMin=[]  FilterOutMax=[]  SumI1OutMin=[]  SumI1OutMax=[]  SumI2OutMin=[]  SumI2OutMax=[]  SumI3OutMin=[]  SumI3OutMax=[]  SumI4OutMin=[]  SumI4OutMax=[]  SumDOutMin=[]  SumDOutMax=[]  DifferentiatorOutMin=[]  DifferentiatorOutMax=[]  FilterDiffOutCoefMin=[]  FilterDiffOutCoefMax=[]  ReciprocalOutMin=[]  ReciprocalOutMax=[]  SumDenOutMin=[]  SumDenOutMax=[]  SumNumOutMin=[]  SumNumOutMax=[]  DivideOutMin=[]  DivideOutMax=[]  UdiffTsProdOutMin=[]  UdiffTsProdOutMax=[]  NTsProdOutMin=[]  NTsProdOutMax=[]  UintegralTsProdOutMin=[]  UintegralTsProdOutMax=[]  UngainTsProdOutMin=[]  UngainTsProdOutMax=[]  ClampingZeroOutDataTypeStr=Inherit: Inherit via back propagation  ClampingZeroOutMin=[]  ClampingZeroOutMax=[]  FilterDenConstantOutDataTypeStr=Inherit: Inherit via back propagation  FilterDenConstantOutMin=[]  FilterDenConstantOutMax=[]  PCopyOutDataTypeStr=Inherit: Inherit via back propagation  PCopyOutMin=[]  PCopyOutMax=[]  NCopyOutDataTypeStr=Inherit: Inherit via back propagation  NCopyOutMin=[]  NCopyOutMax=[]  IntegratorContinuousStateAttributes=''  IntegratorStateMustResolveToSignalObject=off  IntegratorRTWStateStorageClass=Auto  FilterContinuousStateAttributes=''  FilterStateMustResolveToSignalObject=off  FilterRTWStateStorageClass=Auto  ParallelPVariant=InternalParameters  IdealPVariant=Disabled  IVariant=InternalParameters  DVariant=InternalParameters  IntegratorVariant=Discrete  SatVariant=Disabled  AWVariant=Passthrough  PCopyVariant=Disabled  TRVariant=Disabled  FdbkBlocksVariant=Forward  IdealPFdbkVariant=Disabled  SatFdbkVariant=Disabled  DerivativeFilterVariant=ForwardEulerFilter  NVariant=InternalParameters  NCopyVariant=Disabled  FilterICVariant=InternalICsFilter  IntegratorICVariant=InternalICs  ExternalResetVariant=Disabled  TRSumVariant=Passthrough  SumFdbkVariant=Disabled  SumVariant=Sum_PID  TsampFilterVariant=InternalTs  TsampNgainVariant=Passthrough  TsampIntegralVariant=Disabled_SignalSpec  ExternalSaturationOutDataTypeStr=Inherit: Same as second input  DerivativeSourceVariant=ErrorSignal  PreIntVariant=InternalPreInt
  IC : InitialCondition  Value=0
  Sum1 : Sum  Inputs=|+-
  Pitch SP : Outport
  Throttle : Outport  Port=2
  wires:
  IC/1 -> Pitch SP/1
  Pitch SP In/1 -> IC/1
  Airspeed SP/1 -> Sum1/1
  Sum1/1 -> Airspeed Controller/1
  Airspeed/1 -> Sum1/2
  Airspeed Controller/1 -> Throttle/1

== system autocontroller_origin/Auto1/Fixed Wing Controller/Subsystem/Roll SP from Path Manager ==
  In1 : Inport
  Enable : EnablePort
  IC : InitialCondition  Value=0
  Out1 : Outport
  wires:
  In1/1 -> IC/1
  IC/1 -> Out1/1

== system autocontroller_origin/Auto1/Fixed Wing Controller/Subsystem/Subsystem2 ==
  Euler : Inport
  pqr : Inport  Port=2
  Demux : Demux  Outputs=3
  MATLAB Function : MATLAB Function  TreatAsAtomicUnit=on
  Terminator : Terminator
  Terminator1 : Terminator
  Euler Rate : Outport
  wires:
  Demux/1 -> MATLAB Function/1(phi)
  Demux/2 -> MATLAB Function/2(theta)
  MATLAB Function/1(y) -> Terminator1/1
  pqr/1 -> Euler Rate/1
  Euler/1 -> Demux/1
  Demux/3 -> Terminator/1

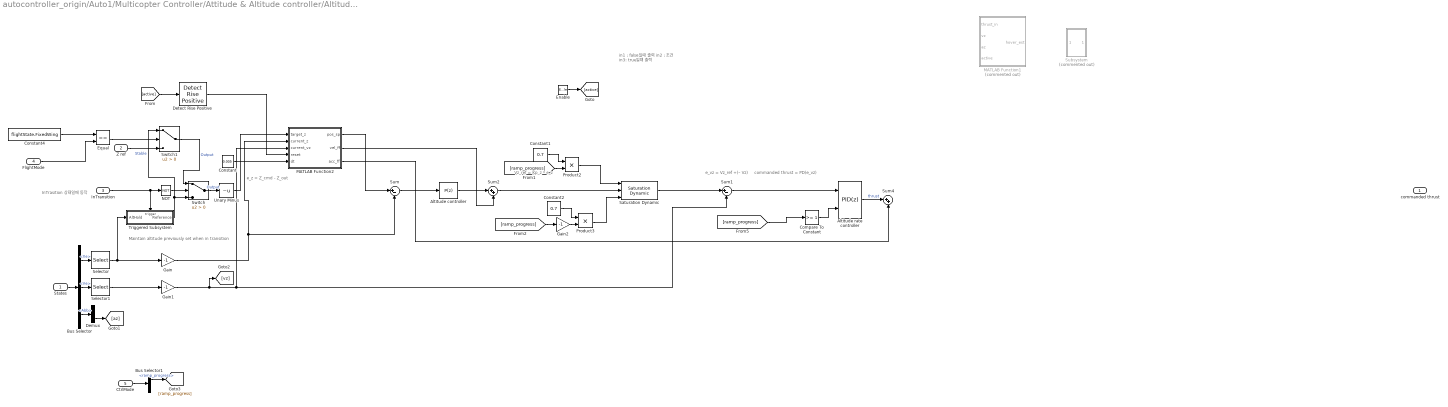
== system autocontroller_origin/Auto1/Multicopter Controller/Attitude & Altitude controller/Altitude Control ==
  note: commanded thrust = PD(e_vz)
  note: e_vz = Vz_ref +(– Vz)
  note: Vz_ref = Kp_z * e_z
  note: e_z = Z_cmd - Z_out
  note: in1 : false일때 출력
      | in2 : 조건
      | in3: true일떄 출력
  note: InTrasition 상태일때 동작
  note: Maintain altitude previously set when in transition
  States : Inport
  Z ref : Inport  Port=2
  InTransition : Inport  Port=3
  FlightMode : Inport  Port=4
  CtrlMode : Inport  Port=5
  Enable : EnablePort  StatesWhenEnabling=reset  ShowOutputPort=on
  Altitude controller : slpidlib/PID Controller  Controller=P  Form=Parallel  TimeDomain=Discrete-time  UseExternalTs=off  SampleTime=-1  IntegratorMethod=Forward Euler  FilterMethod=Forward Euler  ControllerParametersSource=internal  P=controlParams.P_Z  I=controlParams.I_Z  UseKiTs=off  D=controlParams.D_Z  UseExternalDerivativeSource=off  N=controlParams.N_Z  UseFilter=on  TunerSelectOption=Transfer Function Based (PID Tuner App)  InitialConditionSource=internal  InitialConditionForIntegrator=0  InitialConditionForFilter=0  DifferentiatorICPrevScaledInput=0  ExternalReset=none  TrackingMode=off  Kt=1  LimitOutput=on  SatLimitsSource=internal  UpperSaturationLimit=5  LowerSaturationLimit=-5  LinearizeAsGain=on  AntiWindupMode=none  Kb=1  LimitIntegrator=off  UpperIntegratorSaturationLimit=inf  LowerIntegratorSaturationLimit=-inf  POutMin=[]  POutMax=[]  IOutMin=[]  IOutMax=[]  DOutMin=[]  DOutMax=[]  NOutMin=[]  NOutMax=[]  SumOutMin=[]  SumOutMax=[]  SaturationOutMin=[]  SaturationOutMax=[]  PParamMin=[]  PParamMax=[]  IParamMin=[]  IParamMax=[]  DParamMin=[]  DParamMax=[]  NParamMin=[]  NParamMax=[]  KbParamMin=[]  KbParamMax=[]  KtParamMin=[]  KtParamMax=[]  KbOutMin=[]  KbOutMax=[]  KtOutMin=[]  KtOutMax=[]  IntegratorOutMin=[]  IntegratorOutMax=[]  FilterOutMin=[]  FilterOutMax=[]  SumI1OutMin=[]  SumI1OutMax=[]  SumI2OutMin=[]  SumI2OutMax=[]  SumI3OutMin=[]  SumI3OutMax=[]  SumI4OutMin=[]  SumI4OutMax=[]  SumDOutMin=[]  SumDOutMax=[]  DifferentiatorOutMin=[]  DifferentiatorOutMax=[]  FilterDiffOutCoefMin=[]  FilterDiffOutCoefMax=[]  ReciprocalOutMin=[]  ReciprocalOutMax=[]  SumDenOutMin=[]  SumDenOutMax=[]  SumNumOutMin=[]  SumNumOutMax=[]  DivideOutMin=[]  DivideOutMax=[]  UdiffTsProdOutMin=[]  UdiffTsProdOutMax=[]  NTsProdOutMin=[]  NTsProdOutMax=[]  UintegralTsProdOutMin=[]  UintegralTsProdOutMax=[]  UngainTsProdOutMin=[]  UngainTsProdOutMax=[]  ClampingZeroOutDataTypeStr=Inherit: Inherit via back propagation  ClampingZeroOutMin=[]  ClampingZeroOutMax=[]  FilterDenConstantOutDataTypeStr=Inherit: Inherit via back propagation  FilterDenConstantOutMin=[]  FilterDenConstantOutMax=[]  PCopyOutDataTypeStr=Inherit: Inherit via back propagation  PCopyOutMin=[]  PCopyOutMax=[]  NCopyOutDataTypeStr=Inherit: Inherit via back propagation  NCopyOutMin=[]  NCopyOutMax=[]  IntegratorContinuousStateAttributes=''  IntegratorStateMustResolveToSignalObject=off  IntegratorRTWStateStorageClass=Auto  FilterContinuousStateAttributes=''  FilterStateMustResolveToSignalObject=off  FilterRTWStateStorageClass=Auto  ParallelPVariant=InternalParameters  IdealPVariant=Disabled  IVariant=Disabled  DVariant=Disabled  IntegratorVariant=Disabled  SatVariant=Enabled  AWVariant=Disabled  PCopyVariant=Disabled  TRVariant=Disabled  FdbkBlocksVariant=Forward  IdealPFdbkVariant=Disabled  SatFdbkVariant=Disabled  DerivativeFilterVariant=Disabled  NVariant=Disabled  NCopyVariant=Disabled_SignalSpec  FilterICVariant=Disabled  IntegratorICVariant=Disabled  ExternalResetVariant=Disabled  TRSumVariant=Passthrough  SumFdbkVariant=Disabled  SumVariant=Passthrough_P  TsampFilterVariant=InternalTs  TsampNgainVariant=Passthrough  TsampIntegralVariant=Disabled_SignalSpec  ExternalSaturationOutDataTypeStr=Inherit: Same as second input  DerivativeSourceVariant=Disabled  PreIntVariant=InternalPreInt
  Altitude rate controller : slpidlib/PID Controller  Controller=PID  Form=Parallel  TimeDomain=Discrete-time  UseExternalTs=off  SampleTime=-1  IntegratorMethod=Forward Euler  FilterMethod=Forward Euler  ControllerParametersSource=internal  P=controlParams.P_VZ  I=controlParams.I_VZ  UseKiTs=off  D=controlParams.D_VZ  UseExternalDerivativeSource=off  N=controlParams.N_VZ  UseFilter=on  TunerSelectOption=Transfer Function Based (PID Tuner App)  InitialConditionSource=internal  InitialConditionForIntegrator=0  InitialConditionForFilter=0  DifferentiatorICPrevScaledInput=0  ExternalReset=rising  TrackingMode=off  Kt=1  LimitOutput=on  SatLimitsSource=internal  UpperSaturationLimit=2  LowerSaturationLimit=-2  LinearizeAsGain=on  AntiWindupMode=clamping  Kb=1  LimitIntegrator=on  UpperIntegratorSaturationLimit=2  LowerIntegratorSaturationLimit=-1.5  POutMin=[]  POutMax=[]  IOutMin=[]  IOutMax=[]  DOutMin=[]  DOutMax=[]  NOutMin=[]  NOutMax=[]  SumOutMin=[]  SumOutMax=[]  SaturationOutMin=[]  SaturationOutMax=[]  PParamMin=[]  PParamMax=[]  IParamMin=[]  IParamMax=[]  DParamMin=[]  DParamMax=[]  NParamMin=[]  NParamMax=[]  KbParamMin=[]  KbParamMax=[]  KtParamMin=[]  KtParamMax=[]  KbOutMin=[]  KbOutMax=[]  KtOutMin=[]  KtOutMax=[]  IntegratorOutMin=[]  IntegratorOutMax=[]  FilterOutMin=[]  FilterOutMax=[]  SumI1OutMin=[]  SumI1OutMax=[]  SumI2OutMin=[]  SumI2OutMax=[]  SumI3OutMin=[]  SumI3OutMax=[]  SumI4OutMin=[]  SumI4OutMax=[]  SumDOutMin=[]  SumDOutMax=[]  DifferentiatorOutMin=[]  DifferentiatorOutMax=[]  FilterDiffOutCoefMin=[]  FilterDiffOutCoefMax=[]  ReciprocalOutMin=[]  ReciprocalOutMax=[]  SumDenOutMin=[]  SumDenOutMax=[]  SumNumOutMin=[]  SumNumOutMax=[]  DivideOutMin=[]  DivideOutMax=[]  UdiffTsProdOutMin=[]  UdiffTsProdOutMax=[]  NTsProdOutMin=[]  NTsProdOutMax=[]  UintegralTsProdOutMin=[]  UintegralTsProdOutMax=[]  UngainTsProdOutMin=[]  UngainTsProdOutMax=[]  ClampingZeroOutDataTypeStr=Inherit: Inherit via back propagation  ClampingZeroOutMin=[]  ClampingZeroOutMax=[]  FilterDenConstantOutDataTypeStr=Inherit: Inherit via back propagation  FilterDenConstantOutMin=[]  FilterDenConstantOutMax=[]  PCopyOutDataTypeStr=Inherit: Inherit via back propagation  PCopyOutMin=[]  PCopyOutMax=[]  NCopyOutDataTypeStr=Inherit: Inherit via back propagation  NCopyOutMin=[]  NCopyOutMax=[]  IntegratorContinuousStateAttributes=''  IntegratorStateMustResolveToSignalObject=off  IntegratorRTWStateStorageClass=Auto  FilterContinuousStateAttributes=''  FilterStateMustResolveToSignalObject=off  FilterRTWStateStorageClass=Auto  ParallelPVariant=InternalParameters  IdealPVariant=Disabled  IVariant=InternalParameters  DVariant=InternalParameters  IntegratorVariant=Discrete  SatVariant=Enabled  AWVariant=DiscClampingParallel  PCopyVariant=Disabled  TRVariant=Disabled  FdbkBlocksVariant=Forward  IdealPFdbkVariant=Disabled  SatFdbkVariant=Disabled  DerivativeFilterVariant=ForwardEulerFilter  NVariant=InternalParameters  NCopyVariant=Disabled  FilterICVariant=InternalICsFilter  IntegratorICVariant=InternalICs  ExternalResetVariant=ExternalReset  TRSumVariant=Passthrough  SumFdbkVariant=Disabled  SumVariant=Sum_PID  TsampFilterVariant=InternalTs  TsampNgainVariant=Passthrough  TsampIntegralVariant=Disabled_SignalSpec  ExternalSaturationOutDataTypeStr=Inherit: Same as second input  DerivativeSourceVariant=ErrorSignal  PreIntVariant=InternalPreInt
  Bus Selector : BusSelector  OutputSignals=Xe,Ve,Abb
  Bus Selector1 : BusSelector  OutputSignals=ramp_progress,spoolup_active
  Compare To Constant : simulink/Logic and Bit Operations/Compare To Constant  relop=>=  const=1  OutDataTypeStr=boolean
  Constant : Constant  Value=0.005
  Constant1 : Constant  Value=0.7
  Constant2 : Constant  Value=0.7
  Constant4 : Constant  Value=flightState.FixedWing
  Demux : Demux  Outputs=3
  Detect Rise Positive : simulink/Logic and Bit Operations/Detect Rise Positive  vinit=0  OutDataTypeStr=boolean
  Equal : RelationalOperator  Operator===  OutDataTypeStr=boolean  RndMeth=Simplest  InputSameDT=off
  Gain : Gain  Gain=-1
  Gain1 : Gain  Gain=-1
  Gain2 : Gain  Gain=-1
  MATLAB Function1 : MATLAB Function  Commented=on  TreatAsAtomicUnit=on
  MATLAB Function2 : MATLAB Function  TreatAsAtomicUnit=on
  NOT : Logic  Operator=NOT  IconShape=distinctive  AllPortsSameDT=off  OutDataTypeStr=boolean
  Product2 : Product
  Product3 : Product
  Saturation Dynamic : simulink/Discontinuities/Saturation Dynamic  OutMin=[]  OutMax=[]  OutDataTypeStr=Inherit: Same as second input  OutDataType=fixdt(1, 16)  OutScaling=2^-10  DoSatur=off
  Selector : Selector  InputPortWidth=3  IndexOptions=Index vector (dialog)  Indices=[3]  OutputSizes=1
  Selector1 : Selector  InputPortWidth=3  IndexOptions=Index vector (dialog)  Indices=[3]  OutputSizes=1
  Subsystem : Subsystem  Commented=on
  Sum : Sum  Inputs=|+-
  Sum1 : Sum  Inputs=|+-
  Sum2 : Sum  Inputs=|++
  Sum4 : Sum  Inputs=|++
  Switch : Switch  Criteria=u2 > Threshold  SaturateOnIntegerOverflow=off  InputSameDT=off
  Switch1 : Switch  Criteria=u2 > Threshold  SaturateOnIntegerOverflow=off  InputSameDT=off
  Triggered Subsystem : Subsystem  TreatAsAtomicUnit=on
  Unary Minus : UnaryMinus
  commanded thrust : Outport
  wires:
  States/1 -> Bus Selector/1
  InTransition/1 -> NOT/1, Triggered Subsystem/Trigger
  Switch/1 -> Unary Minus/1  "Output"
  NOT/1 -> Switch/2
  Triggered Subsystem/1(Reference) -> Switch1/1, Switch/3  "Stable"
  Bus Selector/1 -> Selector/1  "<Xe>"
  Bus Selector/2 -> Selector1/1  "<Ve>"
  Constant4/1 -> Equal/1
  FlightMode/1 -> Equal/2
  Equal/1 -> Switch1/2
  Z ref/1 -> Switch1/3
  Switch1/1 -> Switch/1  "Output"
  Sum/1 -> Altitude controller/1
  Selector1/1 -> Gain1/1
  Selector/1 -> Gain/1, Triggered Subsystem/1(AltHold)
  Gain/1 -> Sum/2, MATLAB Function2/2(current_z)
  Gain1/1 -> [vz], Sum1/2, MATLAB Function2/3(current_vz)
  Enable/1 -> [active]
  Compare To Constant/1 -> Altitude rate controller/2
  Sum1/1 -> Altitude rate controller/1
  Bus Selector/3 -> Demux/1  "<Abb>"
  Demux/3 -> [az]
  Unary Minus/1 -> MATLAB Function2/1(target_z)
  CtrlMode/1 -> Bus Selector1/1
  Bus Selector1/1 -> [ramp_progress]  "<ramp_progress>"
  [ramp_progress] -> Product2/2
  Constant1/1 -> Product2/1
  Constant2/1 -> Product3/1
  [ramp_progress] -> Gain2/1
  Product3/1 -> Saturation Dynamic/3
  Product2/1 -> Saturation Dynamic/1
  Gain2/1 -> Product3/2
  [ramp_progress] -> Compare To Constant/1
  Constant/1 -> MATLAB Function2/5(dt)
  [active] -> Detect Rise Positive/1
  Detect Rise Positive/1 -> MATLAB Function2/4(reset)
  MATLAB Function2/1(pos_sp) -> Sum/1
  Saturation Dynamic/1 -> Sum1/1
  Altitude controller/1 -> Sum2/1
  Sum2/1 -> Saturation Dynamic/2
  MATLAB Function2/2(vel_ff) -> Sum2/2
  Altitude rate controller/1 -> Sum4/1  "thrust"
  MATLAB Function2/3(acc_ff) -> Sum4/2
